simulink model "calibration"  (R2025b)
settings: Solver=ode5  StartTime=0.0  StopTime=50  RelTol=1e-3
values from neighbouring files (symbols this model uses):
  SampleTime = 0.001    [main_lab.m]
undefined symbols (not defined in the file or in its folder): National_Instruments, PCI
libraries: sldrtlib x6
settings Model: Creator=aie4-26  LastModifiedBy=aie4-26
settings HardwareCC: ProdBitPerLong=64.0  ProdHWDeviceType=Intel->x86-64 (Linux 64)
settings RTWCC: SystemTargetFile=sldrt.tlc  TemplateMakefile=sldrt.tmf  RTWCompilerOptimization=on  Description=Simulink Desktop Real-Time
settings CodeAppCC: MaxIdLength=95.0
settings SimulinkDesktopRealTimeCC: ExtModeTransport=0.0  ExtModeStaticAllocSize=1000000.0  TargetLibSuffix=_sldrt.a  TargetPreCompLibLocation=C:\Program Files\MATLAB\R2025b\toolbox\sldrt\lib\win64  MultiwordLength=2048.0  DynamicStringBufferSize=256.0  ParMdlRefBuildCompliant=on  PreserveMATLABNamespacesInGeneratedCode=on  SubcomponentCodeInterfacePackaging=Reusable function

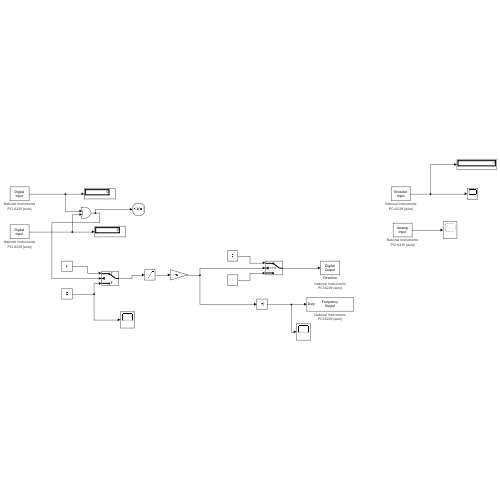
[thumbnail: Simulink's stored preview of the top-level diagram]
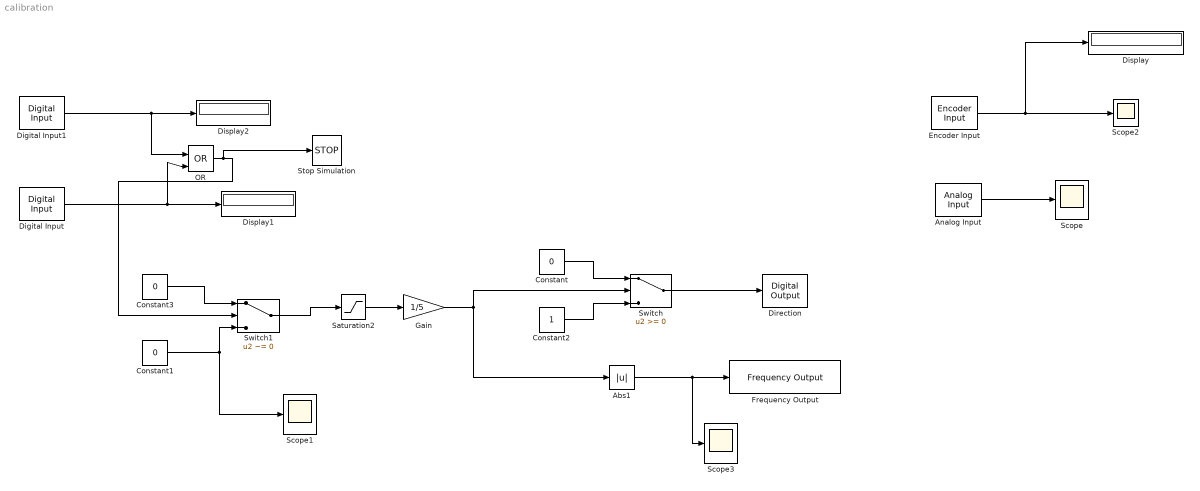
== system calibration ==
  Abs1 : Abs  SaturateOnIntegerOverflow=off
  Analog Input : sldrtlib/Analog Input  SampleTime=SampleTime  MaxMissedTicks=MaxMissedTicks  ShowMissedTicks=off  YieldWhenWaiting=off  DrvName=National_Instruments/PCI-6229  DrvAddress=4294967295  DrvOptions=[1 1 8192 2 3]  Channels=1  RangeMode=1  VoltRange=1  DataType=1
      settings: AttributesFormatString=National Instruments\nPCI-6229 [auto]
  Constant : Constant  Value=0  SampleTime=SampleTime
  Constant1 : Constant  Value=0
  Constant2 : Constant  SampleTime=SampleTime
  Constant3 : Constant  Value=0
  Digital Input : sldrtlib/Digital Input  SampleTime=0.1  MaxMissedTicks=10  ShowMissedTicks=off  YieldWhenWaiting=off  DrvName=National_Instruments/PCI-6229  DrvAddress=4294967295  DrvOptions=[1 1 8192 2 3]  Channels=3  BitMode=1  DataType=9
      settings: AttributesFormatString=National Instruments\nPCI-6229 [auto]
  Digital Input1 : sldrtlib/Digital Input  SampleTime=0.1  MaxMissedTicks=10  ShowMissedTicks=off  YieldWhenWaiting=off  DrvName=National_Instruments/PCI-6229  DrvAddress=4294967295  DrvOptions=[1 1 8192 2 3]  Channels=2  BitMode=1  DataType=9
      settings: AttributesFormatString=National Instruments\nPCI-6229 [auto]
  Direction : sldrtlib/Digital Output  SampleTime=SampleTime  MaxMissedTicks=MaxMissedTicks  ShowMissedTicks=off  YieldWhenWaiting=off  DrvName=National_Instruments/PCI-6229  DrvAddress=4294967295  DrvOptions=[1 1 8192 2 3]  Channels=1  BitMode=1  InitialValue=0  FinalValue=0
      settings: AttributesFormatString=National Instruments\nPCI-6229 [auto]
  Display : Display
  Display1 : Display
  Display2 : Display
  Encoder Input : sldrtlib/Encoder Input  SampleTime=SampleTime  MaxMissedTicks=MaxMissedTicks  ShowMissedTicks=off  YieldWhenWaiting=off  DrvName=National_Instruments/PCI-6229  DrvAddress=4294967295  DrvOptions=[1 1 8192 2 3]  Channels=1  QuadMode=3  IndexPulse=2  InputFilter=Inf  DataType=1
      settings: AttributesFormatString=National Instruments\nPCI-6229 [auto]
  Frequency Output : sldrtlib/Frequency Output  SampleTime=SampleTime  MaxMissedTicks=MaxMissedTicks  ShowMissedTicks=off  YieldWhenWaiting=off  DrvName=National_Instruments/PCI-6229  DrvAddress=4294967295  DrvOptions=[1 1 8192 2 3]  Channels=2  FrequencySource=1  Frequency=10000  FrequencyFinalValue=[]  DutySource=2  Duty=0  DutyFinalValue=0
      settings: AttributesFormatString=National Instruments\nPCI-6229 [auto]
  Gain : Gain  Gain=1/5
  OR : Logic  Operator=OR  IconShape=distinctive  AllPortsSameDT=off  OutDataTypeStr=boolean
  Saturation2 : Saturate  UpperLimit=2.5  LowerLimit=-2.5
  Scope{,1..3} (4 alike) : Scope
      Scope settings: ActiveDisplayYMinimum=0.46535274975515928  ActiveDisplayYMaximum=3.2069525358121433
      Scope1 settings: ActiveDisplayYMinimum=-0.82199195445766415  ActiveDisplayYMaximum=-0.80877401332347065
      Scope2 settings: ActiveDisplayYMinimum=-84.374719376853562  ActiveDisplayYMaximum=0.83932777955028115  DataLoggingVariableName=ScopeData2
      Scope3 settings: ActiveDisplayYMinimum=-1  ActiveDisplayYMaximum=1  DataLoggingVariableName=ScopeData3
  Stop Simulation : Stop
  Switch : Switch  SaturateOnIntegerOverflow=off  InputSameDT=off
  Switch1 : Switch  Criteria=u2 ~= 0  Threshold=1  SaturateOnIntegerOverflow=off  InputSameDT=off
  wires:
  Analog Input/1 -> Scope/1
  Constant/1 -> Switch/1
  Digital Input1/1 -> OR/1, Display2/1
  Abs1/1 -> Scope3/1, Frequency Output/1
  Digital Input/1 -> OR/2, Display1/1
  Saturation2/1 -> Gain/1
  Constant2/1 -> Switch/3
  Encoder Input/1 -> Display/1, Scope2/1
  Switch/1 -> Direction/1
  OR/1 -> Stop Simulation/1, Switch1/2
  Constant3/1 -> Switch1/1
  Switch1/1 -> Saturation2/1
  Gain/1 -> Abs1/1, Switch/2
  Constant1/1 -> Switch1/3, Scope1/1
